simulink model "kre_discrete_observer_wrapper"  (R2026a)
settings: Solver=FixedStepDiscrete  FixedStep=5e-5
settings Model: Creator=hzldx  LastModifiedBy=ASUS
settings HardwareCC: ProdLargestAtomicInteger=Long  ProdLargestAtomicFloat=Double  ProdHWDeviceType=ARM Compatible->ARM Cortex-M  TargetLargestAtomicInteger=Long  TargetLargestAtomicFloat=Double  TargetIntDivRoundTo=Zero  TargetEndianess=LittleEndian  TargetHWDeviceType=ARM Compatible->ARM Cortex-M  ProdEqTarget=off
settings RTWCC: SystemTargetFile=ert.tlc  GenCodeOnly=on  GenerateMakefile=off  Description=Embedded Coder
settings ERTTargetCC: GenerateSampleERTMain=on

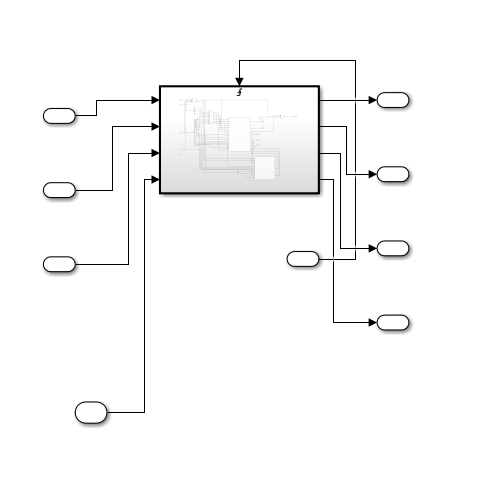
[thumbnail: Simulink's stored preview of the top-level diagram]
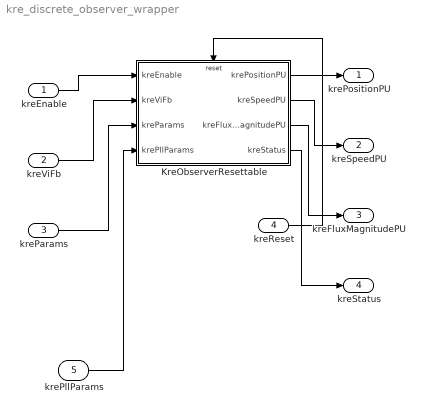
== system kre_discrete_observer_wrapper ==
  kreEnable : Inport  OutDataTypeStr=uint8  PortDimensions=1  SampleTime=5e-5
  kreViFb : Inport  Port=2  OutDataTypeStr=single  PortDimensions=[4 1]  SampleTime=5e-5
  kreParams : Inport  Port=3  OutDataTypeStr=single  PortDimensions=[14 1]  SampleTime=5e-5
  kreReset : Inport  Port=4  OutDataTypeStr=uint8  PortDimensions=1  SampleTime=5e-5
  krePllParams : Inport  Port=5  OutDataTypeStr=single  PortDimensions=[2 1]  SampleTime=5e-5
  KreObserverResettable : Subsystem  TreatAsAtomicUnit=on
  krePositionPU : Outport  OutDataTypeStr=single  PortDimensions=1  SampleTime=5e-5
  kreSpeedPU : Outport  Port=2  OutDataTypeStr=single  PortDimensions=1  SampleTime=5e-5
  kreFluxMagnitudePU : Outport  Port=3  OutDataTypeStr=single  PortDimensions=1  SampleTime=5e-5
  kreStatus : Outport  Port=4  OutDataTypeStr=uint8  PortDimensions=1  SampleTime=5e-5
  wires:
  kreReset/1 -> KreObserverResettable/Reset
  kreEnable/1 -> KreObserverResettable/1(kreEnable)
  kreViFb/1 -> KreObserverResettable/2(kreViFb)
  kreParams/1 -> KreObserverResettable/3(kreParams)
  KreObserverResettable/1(krePositionPU) -> krePositionPU/1
  KreObserverResettable/2(kreSpeedPU) -> kreSpeedPU/1
  KreObserverResettable/3(kreFluxMagnitudePU) -> kreFluxMagnitudePU/1
  KreObserverResettable/4(kreStatus) -> kreStatus/1
  krePllParams/1 -> KreObserverResettable/4(krePllParams)

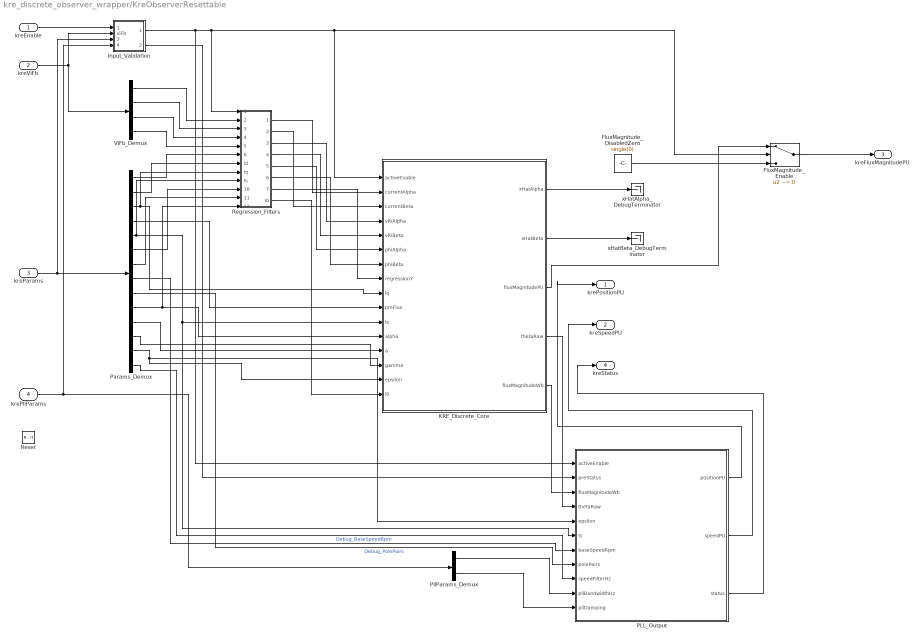
== system kre_discrete_observer_wrapper/KreObserverResettable ==
  kreEnable : Inport  OutDataTypeStr=uint8  PortDimensions=1  SampleTime=5e-5
  kreViFb : Inport  Port=2  OutDataTypeStr=single  PortDimensions=[4 1]  SampleTime=5e-5
  kreParams : Inport  Port=3  OutDataTypeStr=single  PortDimensions=[14 1]  SampleTime=5e-5
  krePllParams : Inport  Port=4  OutDataTypeStr=single  PortDimensions=[2 1]  SampleTime=5e-5
  Reset : ResetPort  DisableCoverage=on
  FluxMagnitude_DisabledZero : Constant  Value=single(0)  OutDataTypeStr=single
  FluxMagnitude_Enable : Switch  Criteria=u2 ~= 0  SaturateOnIntegerOverflow=off  InputSameDT=off
  Input_Validation : Subsystem
  KRE_Discrete_Core : Subsystem
  PLL_Output : Subsystem
  Params_Demux : Demux  Outputs=14
  PllParams_Demux : Demux  Outputs=2
  Regression_Filters : Subsystem
  ViFb_Demux : Demux
  xHatAlpha_DebugTerminator : Terminator
  xHatBeta_DebugTerminator : Terminator
  krePositionPU : Outport  OutDataTypeStr=single  PortDimensions=1  SampleTime=5e-5
  kreSpeedPU : Outport  Port=2  OutDataTypeStr=single  PortDimensions=1  SampleTime=5e-5
  kreFluxMagnitudePU : Outport  Port=3  OutDataTypeStr=single  PortDimensions=1  SampleTime=5e-5
  kreStatus : Outport  Port=4  OutDataTypeStr=uint8  PortDimensions=1  SampleTime=5e-5
  wires:
  Params_Demux/7 -> Regression_Filters/11(baseCurrent)
  Params_Demux/6 -> Regression_Filters/10(baseVoltage)
  Params_Demux/2 -> Regression_Filters/7(ld)
  Params_Demux/1 -> Regression_Filters/6(resistance)
  ViFb_Demux/4 -> Regression_Filters/5(iBetaPU)
  ViFb_Demux/3 -> Regression_Filters/4(iAlphaPU)
  ViFb_Demux/2 -> Regression_Filters/3(vBetaPU)
  ViFb_Demux/1 -> Regression_Filters/2(vAlphaPU)
  kreEnable/1 -> Input_Validation/1(enable)
  kreParams/1 -> Params_Demux/1, Input_Validation/3(params)
  kreViFb/1 -> Input_Validation/2(viFb), ViFb_Demux/1
  KRE_Discrete_Core/2(xHatBeta) -> xHatBeta_DebugTerminator/1
  KRE_Discrete_Core/1(xHatAlpha) -> xHatAlpha_DebugTerminator/1
  Params_Demux/3 -> KRE_Discrete_Core/9(lq), Regression_Filters/8(lq)
  Params_Demux/10 -> KRE_Discrete_Core/12(alpha), Regression_Filters/12(alpha)
  Regression_Filters/1(currentAlpha) -> KRE_Discrete_Core/2(currentAlpha)
  Regression_Filters/2(currentBeta) -> KRE_Discrete_Core/3(currentBeta)
  Regression_Filters/3(vRiAlpha) -> KRE_Discrete_Core/4(vRiAlpha)
  Regression_Filters/4(vRiBeta) -> KRE_Discrete_Core/5(vRiBeta)
  Regression_Filters/5(phiAlpha) -> KRE_Discrete_Core/6(phiAlpha)
  Regression_Filters/6(phiBeta) -> KRE_Discrete_Core/7(phiBeta)
  Regression_Filters/7(regressionY) -> KRE_Discrete_Core/8(regressionY)
  Params_Demux/4 -> KRE_Discrete_Core/10(pmFlux)
  Params_Demux/11 -> KRE_Discrete_Core/13(a)
  Params_Demux/12 -> KRE_Discrete_Core/14(gamma)
  Regression_Filters/8(l0) -> KRE_Discrete_Core/16(l0)
  FluxMagnitude_Enable/1 -> kreFluxMagnitudePU/1
  FluxMagnitude_DisabledZero/1 -> FluxMagnitude_Enable/3
  KRE_Discrete_Core/3(fluxMagnitudePU) -> FluxMagnitude_Enable/1
  PLL_Output/3(status) -> kreStatus/1
  PLL_Output/2(speedPU) -> kreSpeedPU/1
  PLL_Output/1(positionPU) -> krePositionPU/1
  PllParams_Demux/2 -> PLL_Output/11(pllDamping)
  PllParams_Demux/1 -> PLL_Output/10(pllBandwidthHz)
  Params_Demux/14 -> PLL_Output/9(speedFilterHz)
  Params_Demux/9 -> PLL_Output/8(polePairs)  "Debug_PolePairs"
  Params_Demux/8 -> PLL_Output/7(baseSpeedRpm)  "Debug_BaseSpeedRpm"
  KRE_Discrete_Core/4(thetaRaw) -> PLL_Output/4(thetaRaw)
  Input_Validation/2(preStatus) -> PLL_Output/2(preStatus)
  Params_Demux/13 -> KRE_Discrete_Core/15(epsilon), PLL_Output/5(epsilon)
  Params_Demux/5 -> PLL_Output/6(ts), KRE_Discrete_Core/11(ts), Regression_Filters/9(ts)
  Input_Validation/1(activeEnable) -> FluxMagnitude_Enable/2, KRE_Discrete_Core/1(activeEnable), Regression_Filters/1(activeEnable), PLL_Output/1(activeEnable)
  krePllParams/1 -> PllParams_Demux/1, Input_Validation/4(pllParams)
  KRE_Discrete_Core/5(fluxMagnitudeWb) -> PLL_Output/3(fluxMagnitudeWb)

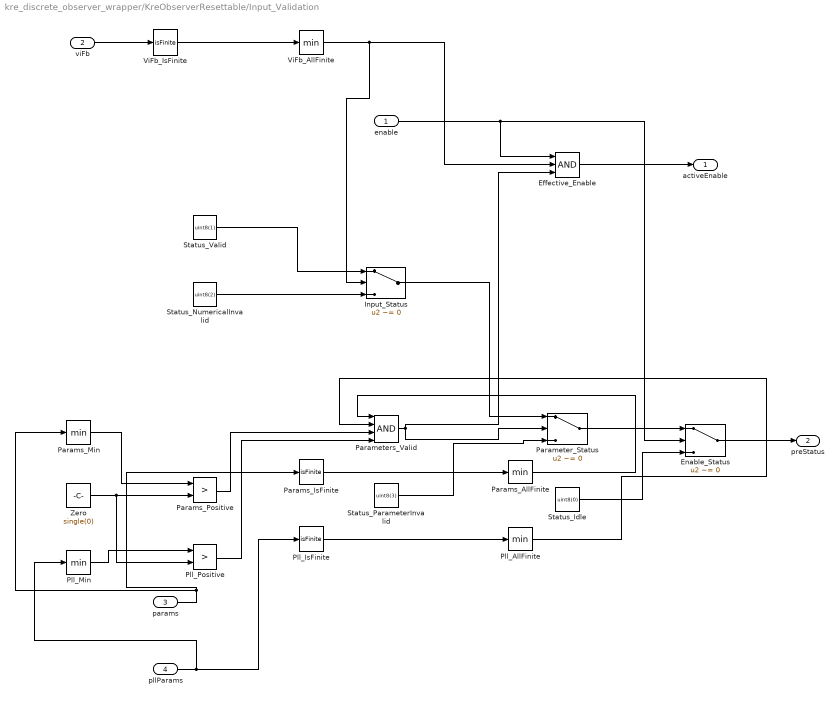
== system kre_discrete_observer_wrapper/KreObserverResettable/Input_Validation ==
  enable : Inport
  viFb : Inport  Port=2
  params : Inport  Port=3
  pllParams : Inport  Port=4
  Effective_Enable : Logic  Inputs=3  IconShape=distinctive  AllPortsSameDT=off  OutDataTypeStr=boolean
  Enable_Status : Switch  Criteria=u2 ~= 0  SaturateOnIntegerOverflow=off  InputSameDT=off
  Input_Status : Switch  Criteria=u2 ~= 0  SaturateOnIntegerOverflow=off  InputSameDT=off
  Parameter_Status : Switch  Criteria=u2 ~= 0  SaturateOnIntegerOverflow=off  InputSameDT=off
  Parameters_Valid : Logic  Inputs=4  IconShape=distinctive  AllPortsSameDT=off  OutDataTypeStr=boolean
  Params_AllFinite : MinMax
  Params_IsFinite : RelationalOperator  Operator=isFinite  OutDataTypeStr=boolean  RndMeth=Simplest  InputSameDT=off
  Params_Min : MinMax
  Params_Positive : RelationalOperator  Operator=>  OutDataTypeStr=boolean  RndMeth=Simplest  InputSameDT=off
  Pll_AllFinite : MinMax
  Pll_IsFinite : RelationalOperator  Operator=isFinite  OutDataTypeStr=boolean  RndMeth=Simplest  InputSameDT=off
  Pll_Min : MinMax
  Pll_Positive : RelationalOperator  Operator=>  OutDataTypeStr=boolean  RndMeth=Simplest  InputSameDT=off
  Status_Idle : Constant  Value=uint8(0)  OutDataTypeStr=uint8
  Status_NumericalInvalid : Constant  Value=uint8(2)  OutDataTypeStr=uint8
  Status_ParameterInvalid : Constant  Value=uint8(3)  OutDataTypeStr=uint8
  Status_Valid : Constant  Value=uint8(1)  OutDataTypeStr=uint8
  ViFb_AllFinite : MinMax
  ViFb_IsFinite : RelationalOperator  Operator=isFinite  OutDataTypeStr=boolean  RndMeth=Simplest  InputSameDT=off
  Zero : Constant  Value=single(0)  OutDataTypeStr=single
  activeEnable : Outport
  preStatus : Outport  Port=2
  wires:
  Enable_Status/1 -> preStatus/1
  Status_Idle/1 -> Enable_Status/3
  Parameter_Status/1 -> Enable_Status/1
  Status_ParameterInvalid/1 -> Parameter_Status/3
  Input_Status/1 -> Parameter_Status/1
  Status_NumericalInvalid/1 -> Input_Status/3
  Status_Valid/1 -> Input_Status/1
  Effective_Enable/1 -> activeEnable/1
  Parameters_Valid/1 -> Effective_Enable/3, Parameter_Status/2
  enable/1 -> Effective_Enable/1, Enable_Status/2
  Pll_Positive/1 -> Parameters_Valid/4
  Params_Positive/1 -> Parameters_Valid/3
  Pll_Min/1 -> Pll_Positive/1
  Zero/1 -> Params_Positive/2, Pll_Positive/2
  Params_Min/1 -> Params_Positive/1
  Pll_IsFinite/1 -> Pll_AllFinite/1
  Params_IsFinite/1 -> Params_AllFinite/1
  ViFb_IsFinite/1 -> ViFb_AllFinite/1
  viFb/1 -> ViFb_IsFinite/1
  params/1 -> Params_IsFinite/1, Params_Min/1
  pllParams/1 -> Pll_IsFinite/1, Pll_Min/1
  Params_AllFinite/1 -> Parameters_Valid/1
  Pll_AllFinite/1 -> Parameters_Valid/2
  ViFb_AllFinite/1 -> Input_Status/2, Effective_Enable/2

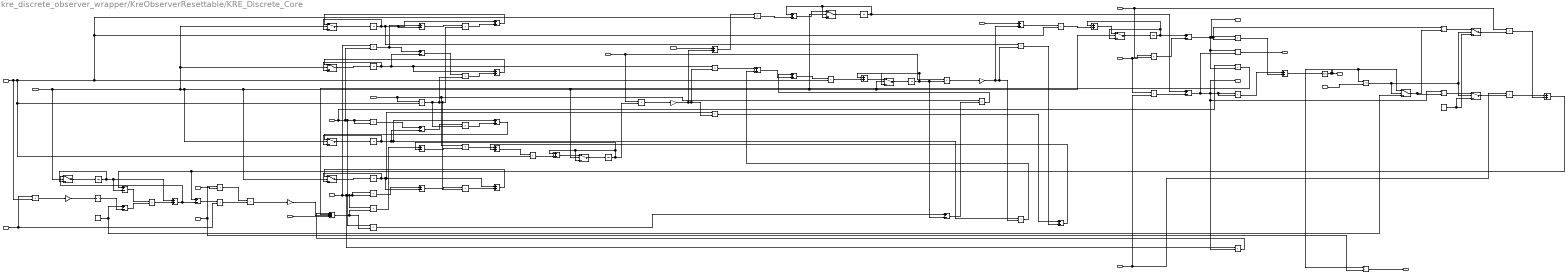
== system kre_discrete_observer_wrapper/KreObserverResettable/KRE_Discrete_Core ==
  activeEnable : Inport
  currentAlpha : Inport  Port=2
  currentBeta : Inport  Port=3
  vRiAlpha : Inport  Port=4
  vRiBeta : Inport  Port=5
  phiAlpha : Inport  Port=6
  phiBeta : Inport  Port=7
  regressionY : Inport  Port=8
  lq : Inport  Port=9
  pmFlux : Inport  Port=10
  ts : Inport  Port=11
  alpha : Inport  Port=12
  a : Inport  Port=13
  gamma : Inport  Port=14
  epsilon : Inport  Port=15
  l0 : Inport  Port=16
  A_Ts : Product
  A_YAlphaError : Product
  A_YBetaError : Product
  ActiveFluxAlpha_Square : Product
  ActiveFluxBeta_Square : Product
  ActiveFlux_Alpha : Sum  Inputs=+-
  ActiveFlux_Beta : Sum  Inputs=+-
  ActiveFlux_Magnitude : Math  Operator=sqrt  SignedPower=on  RndMeth=Zero
  ActiveFlux_NormSquare : Sum
  Alpha_Ts : Product
  CorrectionE_Alpha : Gain  Gain=single(-1)
  CorrectionE_Beta : Gain  Gain=single(-1)
  CurrentDotSigma : Sum
  CurrentDotSigma_Alpha : Product
  CurrentDotSigma_Beta : Product
  Disturbance_Magnitude : Product
  Disturbance_Negative : Gain  Gain=single(-1)
  Exp_NegAlphaTs : Math  SignedPower=on  RndMeth=Zero
  FluxMagnitude_PU : Product  Inputs=*/
  Flux_Above_Epsilon : RelationalOperator  OutDataTypeStr=boolean  RndMeth=Simplest  InputSameDT=off
  Flux_Angle : Trigonometry  Operator=atan2
  GammaY_Alpha : Product
  GammaY_Beta : Product
  H1D : Product
  H1D_Error : Sum  Inputs=+-
  H2D_Correction : Product
  H2D_Error : Sum  Inputs=+-
  H2D_Hold : Switch  Criteria=u2 ~= 0  SaturateOnIntegerOverflow=off  InputSameDT=off
  H2D_Next : Sum
  H2D_State : UnitDelay  InitialCondition=single(0)  SampleTime=-1
  H2_Gain : Sum  Inputs=+-
  LambdaAlpha_Delta : Product
  LambdaAlpha_Derivative : Sum
  LambdaAlpha_Hold : Switch  Criteria=u2 ~= 0  SaturateOnIntegerOverflow=off  InputSameDT=off
  LambdaAlpha_Next : Sum
  LambdaAlpha_State : UnitDelay  InitialCondition=single(0)  SampleTime=-1
  LambdaBeta_Delta : Product
  LambdaBeta_Derivative : Sum
  LambdaBeta_Hold : Switch  Criteria=u2 ~= 0  SaturateOnIntegerOverflow=off  InputSameDT=off
  LambdaBeta_Next : Sum
  LambdaBeta_State : UnitDelay  InitialCondition=single(0)  SampleTime=-1
  Lq_CurrentAlpha : Product
  Lq_CurrentBeta : Product
  Negative_AlphaTs : Gain  Gain=single(-1)
  One : Constant  Value=single(1)  OutDataTypeStr=single
  PhiAlphaBeta : Product
  PhiAlpha_Square : Product
  PhiBeta_Square : Product
  PhiE_Alpha : Product
  PhiE_Beta : Product
  PhiX_Alpha : Product
  PhiX_Beta : Product
  PsiM_L0 : Product
  Q11_Correction : Product
  Q11_EAlpha : Product
  Q11_Hold : Switch  Criteria=u2 ~= 0  SaturateOnIntegerOverflow=off  InputSameDT=off
  Q11_Next : Sum
  Q11_State : UnitDelay  InitialCondition=single(0)  SampleTime=-1
  Q11_TargetMinusState : Sum  Inputs=+-
  Q12_Correction : Product
  Q12_EBeta : Product
  Q12_Hold : Switch  Criteria=u2 ~= 0  SaturateOnIntegerOverflow=off  InputSameDT=off
  Q12_Next : Sum
  Q12_State : UnitDelay  InitialCondition=single(0)  SampleTime=-1
  Q12_TargetMinusState : Sum  Inputs=+-
  Q21_Correction : Product
  Q21_EAlpha : Product
  Q21_Hold : Switch  Criteria=u2 ~= 0  SaturateOnIntegerOverflow=off  InputSameDT=off
  Q21_Next : Sum
  Q21_State : UnitDelay  InitialCondition=single(0)  SampleTime=-1
  Q21_TargetMinusState : Sum  Inputs=+-
  Q22_Correction : Product
  Q22_EBeta : Product
  Q22_Hold : Switch  Criteria=u2 ~= 0  SaturateOnIntegerOverflow=off  InputSameDT=off
  Q22_Next : Sum
  Q22_State : UnitDelay  InitialCondition=single(0)  SampleTime=-1
  Q22_TargetMinusState : Sum  Inputs=+-
  Q_E_Alpha : Sum
  Q_E_Beta : Sum
  Regression_Error : Sum  Inputs=+++-
  Safe_Flux_Magnitude : Switch  Criteria=u2 ~= 0  SaturateOnIntegerOverflow=off  InputSameDT=off
  Sigma_Alpha : Switch  Criteria=u2 ~= 0  SaturateOnIntegerOverflow=off  InputSameDT=off
  Sigma_Alpha_Raw : Product  Inputs=*/
  Sigma_Beta : Switch  Criteria=u2 ~= 0  SaturateOnIntegerOverflow=off  InputSameDT=off
  Sigma_Beta_Raw : Product  Inputs=*/
  YAlpha_Delta : Product
  YAlpha_Derivative : Sum
  YAlpha_Hold : Switch  Criteria=u2 ~= 0  SaturateOnIntegerOverflow=off  InputSameDT=off
  YAlpha_Next : Sum
  YAlpha_State : UnitDelay  InitialCondition=single(0)  SampleTime=-1
  YAlpha_TargetMinusState : Sum  Inputs=+-
  YBeta_Delta : Product
  YBeta_Derivative : Sum
  YBeta_Hold : Switch  Criteria=u2 ~= 0  SaturateOnIntegerOverflow=off  InputSameDT=off
  YBeta_Next : Sum
  YBeta_State : UnitDelay  InitialCondition=single(0)  SampleTime=-1
  YBeta_TargetMinusState : Sum  Inputs=+-
  Zero : Constant  Value=single(0)  OutDataTypeStr=single
  xHatAlpha : Outport
  xHatBeta : Outport  Port=2
  fluxMagnitudePU : Outport  Port=3
  thetaRaw : Outport  Port=4
  fluxMagnitudeWb : Outport  Port=5
  wires:
  Flux_Angle/1 -> thetaRaw/1
  FluxMagnitude_PU/1 -> fluxMagnitudePU/1
  LambdaBeta_Hold/1 -> LambdaBeta_State/1
  LambdaBeta_Next/1 -> LambdaBeta_Hold/1
  LambdaAlpha_Hold/1 -> LambdaAlpha_State/1
  LambdaAlpha_Next/1 -> LambdaAlpha_Hold/1
  LambdaBeta_Delta/1 -> LambdaBeta_Next/2
  LambdaAlpha_Delta/1 -> LambdaAlpha_Next/2
  LambdaBeta_Derivative/1 -> LambdaBeta_Delta/1
  LambdaAlpha_Derivative/1 -> LambdaAlpha_Delta/1
  vRiBeta/1 -> LambdaBeta_Derivative/1
  vRiAlpha/1 -> LambdaAlpha_Derivative/1
  YBeta_Hold/1 -> YBeta_State/1
  YBeta_Next/1 -> YBeta_Hold/1
  YAlpha_Hold/1 -> YAlpha_State/1
  YAlpha_Next/1 -> YAlpha_Hold/1
  YBeta_Delta/1 -> YBeta_Next/2
  YAlpha_Delta/1 -> YAlpha_Next/2
  YBeta_Derivative/1 -> YBeta_Delta/1
  YAlpha_Derivative/1 -> YAlpha_Delta/1
  Q_E_Beta/1 -> YBeta_Derivative/2
  A_YBetaError/1 -> YBeta_Derivative/1
  Q_E_Alpha/1 -> YAlpha_Derivative/2
  A_YAlphaError/1 -> YAlpha_Derivative/1
  YBeta_TargetMinusState/1 -> A_YBetaError/2
  YAlpha_TargetMinusState/1 -> A_YAlphaError/2
  PhiE_Beta/1 -> YBeta_TargetMinusState/1
  PhiE_Alpha/1 -> YAlpha_TargetMinusState/1
  Regression_Error/1 -> PhiE_Alpha/2, PhiE_Beta/2
  Q22_EBeta/1 -> Q_E_Beta/2
  Q21_EAlpha/1 -> Q_E_Beta/1
  Q12_EBeta/1 -> Q_E_Alpha/2
  Q11_EAlpha/1 -> Q_E_Alpha/1
  CorrectionE_Beta/1 -> Q12_EBeta/2, Q22_EBeta/2, LambdaBeta_Derivative/2
  CorrectionE_Alpha/1 -> Q11_EAlpha/2, Q21_EAlpha/2, LambdaAlpha_Derivative/2
  Q22_Hold/1 -> Q22_State/1
  Q22_Next/1 -> Q22_Hold/1
  Q22_Correction/1 -> Q22_Next/2
  Q22_TargetMinusState/1 -> Q22_Correction/1
  Q22_State/1 -> Q22_Next/1, Q22_EBeta/1, Q22_TargetMinusState/2, Q22_Hold/3
  PhiBeta_Square/1 -> Q22_TargetMinusState/1
  Q12_Hold/1 -> Q12_State/1
  Q12_Next/1 -> Q12_Hold/1
  Q12_Correction/1 -> Q12_Next/2
  Q12_TargetMinusState/1 -> Q12_Correction/1
  Q12_State/1 -> Q12_Next/1, Q12_TargetMinusState/2, Q12_EBeta/1, Q12_Hold/3
  Q21_Hold/1 -> Q21_State/1
  Q21_Next/1 -> Q21_Hold/1
  Q21_Correction/1 -> Q21_Next/2
  Q21_TargetMinusState/1 -> Q21_Correction/1
  Q21_State/1 -> Q21_Next/1, Q21_EAlpha/1, Q21_TargetMinusState/2, Q21_Hold/3
  PhiAlphaBeta/1 -> Q21_TargetMinusState/1, Q12_TargetMinusState/1
  Q11_Hold/1 -> Q11_State/1
  Q11_Next/1 -> Q11_Hold/1
  Q11_Correction/1 -> Q11_Next/2
  A_Ts/1 -> Q11_Correction/2, Q12_Correction/2, Q21_Correction/2, Q22_Correction/2
  Q11_TargetMinusState/1 -> Q11_Correction/1
  Q11_State/1 -> Q11_Next/1, Q11_EAlpha/1, Q11_TargetMinusState/2, Q11_Hold/3
  PhiAlpha_Square/1 -> Q11_TargetMinusState/1
  a/1 -> A_YAlphaError/1, A_YBetaError/1, A_Ts/1
  GammaY_Beta/1 -> CorrectionE_Beta/1
  GammaY_Alpha/1 -> CorrectionE_Alpha/1
  YBeta_State/1 -> YBeta_TargetMinusState/2, GammaY_Beta/2, YBeta_Next/1, YBeta_Hold/3
  YAlpha_State/1 -> YAlpha_Next/1, YAlpha_Hold/3, YAlpha_TargetMinusState/2, GammaY_Alpha/2
  gamma/1 -> GammaY_Alpha/1, GammaY_Beta/1
  regressionY/1 -> Regression_Error/4
  Disturbance_Negative/1 -> Regression_Error/3
  PhiX_Beta/1 -> Regression_Error/2
  PhiX_Alpha/1 -> Regression_Error/1
  phiBeta/1 -> PhiBeta_Square/2, PhiBeta_Square/1, PhiE_Beta/1, PhiAlphaBeta/2, PhiX_Beta/1
  phiAlpha/1 -> PhiAlpha_Square/1, PhiAlpha_Square/2, PhiE_Alpha/1, PhiX_Alpha/1, PhiAlphaBeta/1
  Disturbance_Magnitude/1 -> Disturbance_Negative/1
  H1D/1 -> Disturbance_Magnitude/2
  PsiM_L0/1 -> Disturbance_Magnitude/1
  l0/1 -> PsiM_L0/2
  pmFlux/1 -> PsiM_L0/1, FluxMagnitude_PU/2
  H1D_Error/1 -> H1D/1
  H2D_Hold/1 -> H2D_State/1
  activeEnable/1 -> YBeta_Hold/2, LambdaBeta_Hold/2, LambdaAlpha_Hold/2, YAlpha_Hold/2, Q11_Hold/2, Q22_Hold/2, Q21_Hold/2, Q12_Hold/2, H2D_Hold/2
  H2D_Next/1 -> H2D_Hold/1, H1D_Error/2
  H2D_Correction/1 -> H2D_Next/2
  H2_Gain/1 -> H2D_Correction/2
  H2D_Error/1 -> H2D_Correction/1
  H2D_State/1 -> H2D_Error/2, H2D_Next/1, H2D_Hold/3
  CurrentDotSigma/1 -> H2D_Error/1, H1D_Error/1
  CurrentDotSigma_Beta/1 -> CurrentDotSigma/2
  CurrentDotSigma_Alpha/1 -> CurrentDotSigma/1
  Sigma_Beta/1 -> CurrentDotSigma_Beta/2
  Sigma_Alpha/1 -> CurrentDotSigma_Alpha/2
  Sigma_Beta_Raw/1 -> Sigma_Beta/1
  Zero/1 -> Sigma_Alpha/3, Sigma_Beta/3
  Sigma_Alpha_Raw/1 -> Sigma_Alpha/1
  Safe_Flux_Magnitude/1 -> Sigma_Alpha_Raw/2, Sigma_Beta_Raw/2
  Flux_Above_Epsilon/1 -> Sigma_Alpha/2, Sigma_Beta/2, Safe_Flux_Magnitude/2
  epsilon/1 -> Flux_Above_Epsilon/2
  ActiveFlux_NormSquare/1 -> ActiveFlux_Magnitude/1
  ActiveFluxBeta_Square/1 -> ActiveFlux_NormSquare/2
  ActiveFluxAlpha_Square/1 -> ActiveFlux_NormSquare/1
  ActiveFlux_Beta/1 -> Flux_Angle/1, PhiX_Beta/2, Sigma_Beta_Raw/1, ActiveFluxBeta_Square/2, ActiveFluxBeta_Square/1, xHatBeta/1
  ActiveFlux_Alpha/1 -> PhiX_Alpha/2, Sigma_Alpha_Raw/1, ActiveFluxAlpha_Square/2, ActiveFluxAlpha_Square/1, xHatAlpha/1, Flux_Angle/2
  Lq_CurrentBeta/1 -> ActiveFlux_Beta/2
  LambdaBeta_State/1 -> LambdaBeta_Next/1, LambdaBeta_Hold/3, ActiveFlux_Beta/1
  Lq_CurrentAlpha/1 -> ActiveFlux_Alpha/2
  LambdaAlpha_State/1 -> LambdaAlpha_Next/1, LambdaAlpha_Hold/3, ActiveFlux_Alpha/1
  currentBeta/1 -> Lq_CurrentBeta/2, CurrentDotSigma_Beta/1
  currentAlpha/1 -> Lq_CurrentAlpha/2, CurrentDotSigma_Alpha/1
  lq/1 -> Lq_CurrentAlpha/1, Lq_CurrentBeta/1
  Exp_NegAlphaTs/1 -> H2_Gain/2
  One/1 -> H2_Gain/1, Safe_Flux_Magnitude/3
  Negative_AlphaTs/1 -> Exp_NegAlphaTs/1
  Alpha_Ts/1 -> Negative_AlphaTs/1
  ts/1 -> A_Ts/2, YAlpha_Delta/2, LambdaAlpha_Delta/2, LambdaBeta_Delta/2, YBeta_Delta/2, Alpha_Ts/2
  alpha/1 -> Alpha_Ts/1, H1D/2
  ActiveFlux_Magnitude/1 -> Safe_Flux_Magnitude/1, Flux_Above_Epsilon/1, fluxMagnitudeWb/1, FluxMagnitude_PU/1

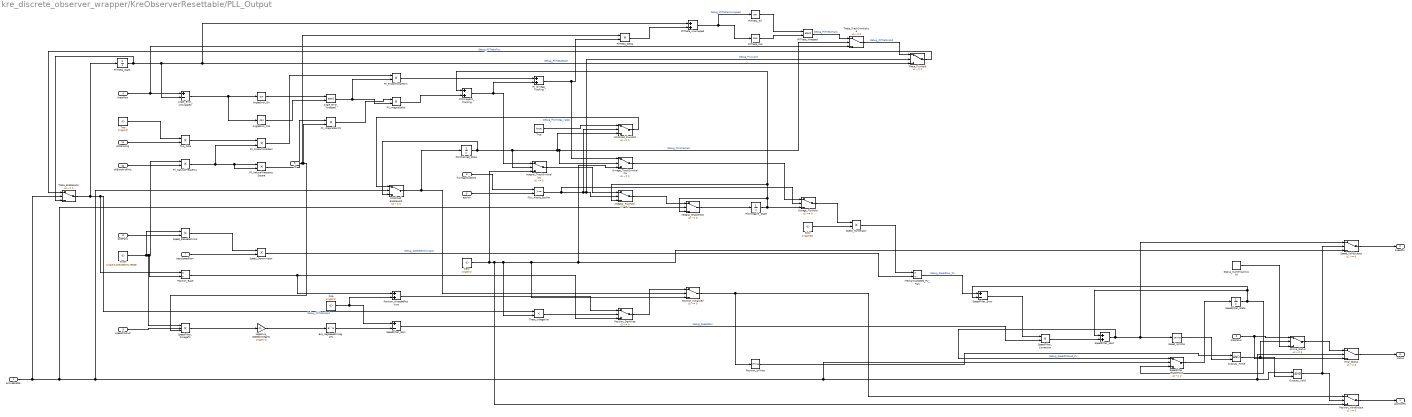
== system kre_discrete_observer_wrapper/KreObserverResettable/PLL_Output ==
  activeEnable : Inport
  preStatus : Inport  Port=2
  fluxMagnitudeWb : Inport  Port=3
  thetaRaw : Inport  Port=4
  epsilon : Inport  Port=5
  ts : Inport  Port=6
  baseSpeedRpm : Inport  Port=7
  polePairs : Inport  Port=8
  speedFilterHz : Inport  Port=9
  pllBandwidthHz : Inport  Port=10
  pllDamping : Inport  Port=11
  Active_Status : Switch  Criteria=u2 ~= 0  SaturateOnIntegerOverflow=off  InputSameDT=off
  AngleError_Cos : Trigonometry  Operator=cos
  AngleError_Sin : Trigonometry
  Angle_Error_Unwrapped : Sum  Inputs=+-
  Angle_Error_Wrapped : Trigonometry  Operator=atan2
  Exp_NegSpeedOmegaTs : Math  SignedPower=on  RndMeth=Zero
  Final_Status : Switch  Criteria=u2 ~= 0  SaturateOnIntegerOverflow=off  InputSameDT=off
  Flux_Above_Epsilon : RelationalOperator  OutDataTypeStr=boolean  RndMeth=Simplest  InputSameDT=off
  Initialized_EnableHold : Switch  Criteria=u2 ~= 0  SaturateOnIntegerOverflow=off  InputSameDT=off
  Initialized_FluxHold : Switch  Criteria=u2 ~= 0  SaturateOnIntegerOverflow=off  InputSameDT=off
  Integral_EnableHold : Switch  Criteria=u2 ~= 0  SaturateOnIntegerOverflow=off  InputSameDT=off
  Integral_FluxHold : Switch  Criteria=u2 ~= 0  SaturateOnIntegerOverflow=off  InputSameDT=off
  Integral_TrackOrInitialize : Switch  Criteria=u2 ~= 0  SaturateOnIntegerOverflow=off  InputSameDT=off
  MechanicalSpeed_PU_Raw : Product  Inputs=*/
  Negative_SpeedOmegaTs : Gain  Gain=single(-1)
  Omega_FluxHold : Switch  Criteria=u2 ~= 0  SaturateOnIntegerOverflow=off  InputSameDT=off
  Omega_TrackOrInitialize : Switch  Criteria=u2 ~= 0  SaturateOnIntegerOverflow=off  InputSameDT=off
  One : Constant  Value=single(1)  OutDataTypeStr=single
  Outputs_Finite : Logic  IconShape=distinctive  AllPortsSameDT=off  OutDataTypeStr=boolean
  Outputs_Valid : Logic  IconShape=distinctive  AllPortsSameDT=off  OutDataTypeStr=boolean
  PllInitialized_State : UnitDelay  InitialCondition=false  SampleTime=-1
  PllOmegaInt_State : UnitDelay  InitialCondition=single(0)  SampleTime=-1
  PllOmegaInt_Tracking : Sum
  PllTheta_Cos : Trigonometry  Operator=cos
  PllTheta_Delta : Product
  PllTheta_Sin : Trigonometry
  PllTheta_State : UnitDelay  InitialCondition=single(0)  SampleTime=-1
  PllTheta_Unwrapped : Sum
  PllTheta_Wrapped : Trigonometry  Operator=atan2
  Pll_IntegralDelta : Product
  Pll_IntegralGainTs : Product
  Pll_NaturalFrequency : Product
  Pll_NaturalFrequencySquare : Product
  Pll_Omega_Tracking : Sum
  Pll_ProportionalGain : Product
  Pll_ProportionalTerm : Product
  Position_Base : Product  Inputs=*/
  Position_Initialized : Switch  Criteria=u2 ~= 0  SaturateOnIntegerOverflow=off  InputSameDT=off
  Position_IsFinite : RelationalOperator  Operator=isFinite  OutDataTypeStr=boolean  RndMeth=Simplest  InputSameDT=off
  Position_SignWrap : Switch  Criteria=u2 ~= 0  SaturateOnIntegerOverflow=off  InputSameDT=off
  Position_ValidOutput : Switch  Criteria=u2 ~= 0  SaturateOnIntegerOverflow=off  InputSameDT=off
  Position_WrappedPositive : Sum
  Sixty : Constant  Value=single(60)  OutDataTypeStr=single
  SpeedFilter_Correction : Product
  SpeedFilter_EnableHold : Switch  Criteria=u2 ~= 0  SaturateOnIntegerOverflow=off  InputSameDT=off
  SpeedFilter_Error : Sum  Inputs=+-
  SpeedFilter_Gain : Sum  Inputs=+-
  SpeedFilter_Next : Sum
  SpeedFilter_OmegaTs : Product  Inputs=***
  SpeedFilter_State : UnitDelay  InitialCondition=single(0)  SampleTime=-1
  Speed_BaseElectrical : Product
  Speed_Denominator : Product
  Speed_IsFinite : RelationalOperator  Operator=isFinite  OutDataTypeStr=boolean  RndMeth=Simplest  InputSameDT=off
  Speed_Numerator : Product
  Speed_ValidOutput : Switch  Criteria=u2 ~= 0  SaturateOnIntegerOverflow=off  InputSameDT=off
  Status_NumericalInvalid : Constant  Value=uint8(2)  OutDataTypeStr=uint8
  Theta_EnableHold : Switch  Criteria=u2 ~= 0  SaturateOnIntegerOverflow=off  InputSameDT=off
  Theta_FluxHold : Switch  Criteria=u2 ~= 0  SaturateOnIntegerOverflow=off  InputSameDT=off
  Theta_IsNegative : RelationalOperator  Operator=<  OutDataTypeStr=boolean  RndMeth=Simplest  InputSameDT=off
  Theta_TrackOrInitialize : Switch  Criteria=u2 ~= 0  SaturateOnIntegerOverflow=off  InputSameDT=off
  True : Constant  Value=true  OutDataTypeStr=boolean
  Two : Constant  Value=single(2)  OutDataTypeStr=single
  TwoPi : Constant  Value=single(6.283185307179586)  OutDataTypeStr=single
  Two_Zeta : Product
  Zero : Constant  Value=single(0)  OutDataTypeStr=single
  positionPU : Outport
  speedPU : Outport  Port=2
  status : Outport  Port=3
  wires:
  Final_Status/1 -> status/1
  Speed_ValidOutput/1 -> speedPU/1
  Position_ValidOutput/1 -> positionPU/1
  Active_Status/1 -> Final_Status/1
  Status_NumericalInvalid/1 -> Active_Status/3
  preStatus/1 -> Active_Status/1, Final_Status/3
  Outputs_Valid/1 -> Position_ValidOutput/2, Speed_ValidOutput/2
  Outputs_Finite/1 -> Outputs_Valid/2, Active_Status/2
  Speed_IsFinite/1 -> Outputs_Finite/2
  Position_IsFinite/1 -> Outputs_Finite/1
  Position_Initialized/1 -> Position_IsFinite/1, Position_ValidOutput/1
  Position_SignWrap/1 -> Position_Initialized/1
  Theta_IsNegative/1 -> Position_SignWrap/2
  Position_WrappedPositive/1 -> Position_SignWrap/1
  Position_Base/1 -> Position_WrappedPositive/1, Position_SignWrap/3
  SpeedFilter_EnableHold/1 -> SpeedFilter_State/1
  SpeedFilter_Next/1 -> Speed_IsFinite/1, Speed_ValidOutput/1, SpeedFilter_EnableHold/1  "Debug_SpeedFiltered_PU"
  SpeedFilter_Correction/1 -> SpeedFilter_Next/2
  SpeedFilter_Gain/1 -> SpeedFilter_Correction/2  "Debug_SpeedGain"
  SpeedFilter_Error/1 -> SpeedFilter_Correction/1
  SpeedFilter_State/1 -> SpeedFilter_Error/2, SpeedFilter_Next/1, SpeedFilter_EnableHold/3
  MechanicalSpeed_PU_Raw/1 -> SpeedFilter_Error/1  "Debug_SpeedRaw_PU"
  Exp_NegSpeedOmegaTs/1 -> SpeedFilter_Gain/2
  One/1 -> SpeedFilter_Gain/1, Position_WrappedPositive/2
  Negative_SpeedOmegaTs/1 -> Exp_NegSpeedOmegaTs/1
  SpeedFilter_OmegaTs/1 -> Negative_SpeedOmegaTs/1
  speedFilterHz/1 -> SpeedFilter_OmegaTs/2
  Speed_Denominator/1 -> MechanicalSpeed_PU_Raw/2  "Debug_SpeedDenominator"
  Speed_Numerator/1 -> MechanicalSpeed_PU_Raw/1
  baseSpeedRpm/1 -> Speed_Denominator/2
  Speed_BaseElectrical/1 -> Speed_Denominator/1
  polePairs/1 -> Speed_BaseElectrical/2
  Sixty/1 -> Speed_Numerator/2
  Omega_FluxHold/1 -> Speed_Numerator/1
  Initialized_EnableHold/1 -> PllInitialized_State/1, Position_Initialized/2
  Initialized_FluxHold/1 -> Initialized_EnableHold/1
  Integral_EnableHold/1 -> PllOmegaInt_State/1
  Integral_FluxHold/1 -> Integral_EnableHold/1
  Theta_EnableHold/1 -> Position_Base/1, Theta_IsNegative/1, PllTheta_State/1  "Debug_PllThetaNext"
  activeEnable/1 -> Outputs_Valid/1, Final_Status/2, SpeedFilter_EnableHold/2, Initialized_EnableHold/2, Integral_EnableHold/2, Theta_EnableHold/2
  Theta_FluxHold/1 -> Theta_EnableHold/1  "Debug_PllThetaFlux"
  True/1 -> Initialized_FluxHold/1
  Omega_TrackOrInitialize/1 -> Omega_FluxHold/1
  Integral_TrackOrInitialize/1 -> Integral_FluxHold/1
  Flux_Above_Epsilon/1 -> Theta_FluxHold/2, Integral_FluxHold/2, Initialized_FluxHold/2, Omega_FluxHold/2  "Debug_FluxValid"
  Theta_TrackOrInitialize/1 -> Theta_FluxHold/1  "Debug_PllThetaValid"
  Zero/1 -> Omega_TrackOrInitialize/3, Speed_ValidOutput/3, Position_Initialized/3, Theta_IsNegative/2, Position_ValidOutput/3, Integral_TrackOrInitialize/3
  PllInitialized_State/1 -> Theta_TrackOrInitialize/2, Omega_TrackOrInitialize/2, Initialized_FluxHold/3, Integral_TrackOrInitialize/2, Initialized_EnableHold/3  "Debug_PllInitialized"
  PllTheta_Wrapped/1 -> Theta_TrackOrInitialize/1  "Debug_PllThetaTrack"
  PllTheta_Cos/1 -> PllTheta_Wrapped/2
  PllTheta_Sin/1 -> PllTheta_Wrapped/1
  PllTheta_Unwrapped/1 -> PllTheta_Sin/1, PllTheta_Cos/1  "Debug_PllThetaUnwrapped"
  PllTheta_Delta/1 -> PllTheta_Unwrapped/2
  Pll_Omega_Tracking/1 -> PllTheta_Delta/2, Omega_TrackOrInitialize/1  "Debug_PllOmega_radps"
  PllOmegaInt_Tracking/1 -> Pll_Omega_Tracking/2, Integral_TrackOrInitialize/1
  Pll_ProportionalTerm/1 -> Pll_Omega_Tracking/1
  Pll_ProportionalGain/1 -> Pll_ProportionalTerm/1
  Two_Zeta/1 -> Pll_ProportionalGain/1
  pllDamping/1 -> Two_Zeta/2
  Two/1 -> Two_Zeta/1
  Pll_IntegralDelta/1 -> PllOmegaInt_Tracking/2
  PllOmegaInt_State/1 -> PllOmegaInt_Tracking/1, Integral_FluxHold/3, Integral_EnableHold/3, Omega_FluxHold/3
  Angle_Error_Wrapped/1 -> Pll_IntegralDelta/2, Pll_ProportionalTerm/2
  Pll_IntegralGainTs/1 -> Pll_IntegralDelta/1
  Pll_NaturalFrequencySquare/1 -> Pll_IntegralGainTs/1
  Pll_NaturalFrequency/1 -> Pll_NaturalFrequencySquare/1, Pll_NaturalFrequencySquare/2, Pll_ProportionalGain/2
  pllBandwidthHz/1 -> Pll_NaturalFrequency/2
  TwoPi/1 -> Pll_NaturalFrequency/1, Position_Base/2, SpeedFilter_OmegaTs/1, Speed_BaseElectrical/1
  AngleError_Cos/1 -> Angle_Error_Wrapped/2
  AngleError_Sin/1 -> Angle_Error_Wrapped/1
  Angle_Error_Unwrapped/1 -> AngleError_Sin/1, AngleError_Cos/1
  PllTheta_State/1 -> PllTheta_Unwrapped/1, Theta_FluxHold/3, Angle_Error_Unwrapped/2, Theta_EnableHold/3  "Debug_PllThetaState"
  thetaRaw/1 -> Theta_TrackOrInitialize/3, Angle_Error_Unwrapped/1
  epsilon/1 -> Flux_Above_Epsilon/2
  fluxMagnitudeWb/1 -> Flux_Above_Epsilon/1
  ts/1 -> SpeedFilter_OmegaTs/3, Pll_IntegralGainTs/2, PllTheta_Delta/1

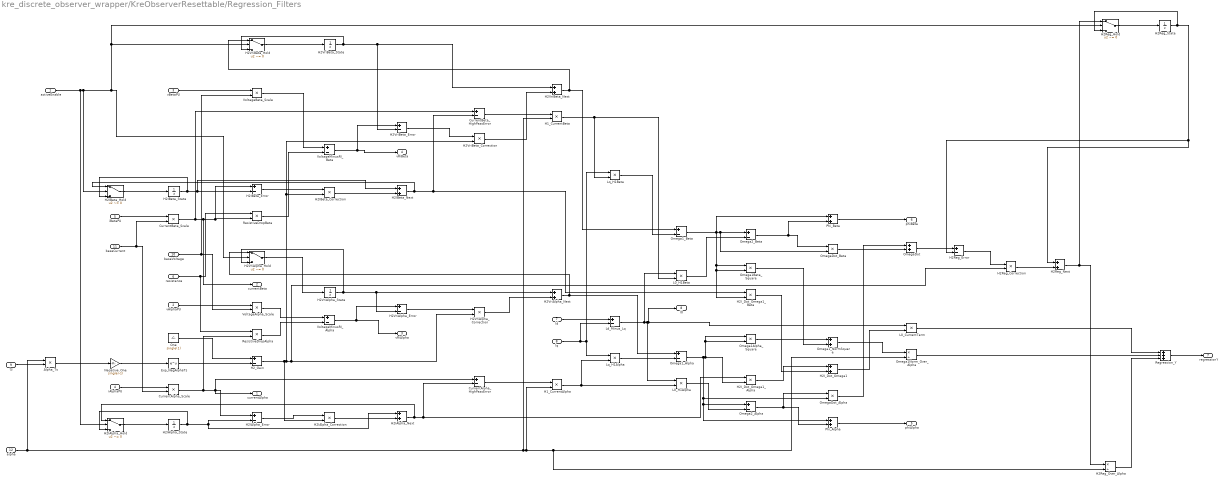
== system kre_discrete_observer_wrapper/KreObserverResettable/Regression_Filters ==
  activeEnable : Inport
  vAlphaPU : Inport  Port=2
  vBetaPU : Inport  Port=3
  iAlphaPU : Inport  Port=4
  iBetaPU : Inport  Port=5
  resistance : Inport  Port=6
  ld : Inport  Port=7
  lq : Inport  Port=8
  ts : Inport  Port=9
  baseVoltage : Inport  Port=10
  baseCurrent : Inport  Port=11
  alpha : Inport  Port=12
  Alpha_Ts : Product
  CurrentAlpha_HighPassError : Sum  Inputs=+-
  CurrentAlpha_Scale : Product
  CurrentBeta_HighPassError : Sum  Inputs=+-
  CurrentBeta_Scale : Product
  Exp_NegAlphaTs : Math  SignedPower=on  RndMeth=Zero
  H1_CurrentAlpha : Product
  H1_CurrentBeta : Product
  H2IAlpha_Correction : Product
  H2IAlpha_Error : Sum  Inputs=+-
  H2IAlpha_Hold : Switch  Criteria=u2 ~= 0  SaturateOnIntegerOverflow=off  InputSameDT=off
  H2IAlpha_Next : Sum
  H2IAlpha_State : UnitDelay  InitialCondition=single(0)  SampleTime=-1
  H2IBeta_Correction : Product
  H2IBeta_Error : Sum  Inputs=+-
  H2IBeta_Hold : Switch  Criteria=u2 ~= 0  SaturateOnIntegerOverflow=off  InputSameDT=off
  H2IBeta_Next : Sum
  H2IBeta_State : UnitDelay  InitialCondition=single(0)  SampleTime=-1
  H2I_Dot_Omega1 : Sum
  H2I_Dot_Omega1_Alpha : Product
  H2I_Dot_Omega1_Beta : Product
  H2Reg_Correction : Product
  H2Reg_Error : Sum  Inputs=+-
  H2Reg_Hold : Switch  Criteria=u2 ~= 0  SaturateOnIntegerOverflow=off  InputSameDT=off
  H2Reg_Next : Sum
  H2Reg_Over_Alpha : Product  Inputs=*/
  H2Reg_State : UnitDelay  InitialCondition=single(0)  SampleTime=-1
  H2VriAlpha_Correction : Product
  H2VriAlpha_Error : Sum  Inputs=+-
  H2VriAlpha_Hold : Switch  Criteria=u2 ~= 0  SaturateOnIntegerOverflow=off  InputSameDT=off
  H2VriAlpha_Next : Sum
  H2VriAlpha_State : UnitDelay  InitialCondition=single(0)  SampleTime=-1
  H2VriBeta_Correction : Product
  H2VriBeta_Error : Sum  Inputs=+-
  H2VriBeta_Hold : Switch  Criteria=u2 ~= 0  SaturateOnIntegerOverflow=off  InputSameDT=off
  H2VriBeta_Next : Sum
  H2VriBeta_State : UnitDelay  InitialCondition=single(0)  SampleTime=-1
  H2_Gain : Sum  Inputs=+-
  L0_CurrentTerm : Product
  L0_H1Alpha : Product
  L0_H1Beta : Product
  Ld_Minus_Lq : Sum  Inputs=+-
  Lq_H1Alpha : Product
  Lq_H1Beta : Product
  Negative_One : Gain  Gain=single(-1)
  Omega1Alpha_Square : Product
  Omega1Beta_Square : Product
  Omega1Norm_Over_Alpha : Product  Inputs=*/
  Omega1_Alpha : Sum  Inputs=+-
  Omega1_Beta : Sum  Inputs=+-
  Omega1_NormSquare : Sum
  Omega2_Alpha : Sum  Inputs=+-
  Omega2_Beta : Sum  Inputs=+-
  OmegaDot : Sum
  OmegaDot_Alpha : Product
  OmegaDot_Beta : Product
  One : Constant  Value=single(1)  OutDataTypeStr=single
  Phi_Alpha : Sum
  Phi_Beta : Sum
  Regression_Y : Sum  Inputs=+++
  ResistiveDropAlpha : Product
  ResistiveDropBeta : Product
  VoltageAlpha_Scale : Product
  VoltageBeta_Scale : Product
  VoltageMinusRI_Alpha : Sum  Inputs=+-
  VoltageMinusRI_Beta : Sum  Inputs=+-
  currentAlpha : Outport
  currentBeta : Outport  Port=2
  vRiAlpha : Outport  Port=3
  vRiBeta : Outport  Port=4
  phiAlpha : Outport  Port=5
  phiBeta : Outport  Port=6
  regressionY : Outport  Port=7
  l0 : Outport  Port=8
  wires:
  Regression_Y/1 -> regressionY/1
  Phi_Beta/1 -> phiBeta/1
  Phi_Alpha/1 -> phiAlpha/1
  H2Reg_Over_Alpha/1 -> Regression_Y/3
  Omega1Norm_Over_Alpha/1 -> Regression_Y/2
  L0_CurrentTerm/1 -> Regression_Y/1
  Omega1_NormSquare/1 -> Omega1Norm_Over_Alpha/1
  Omega1Beta_Square/1 -> Omega1_NormSquare/2
  Omega1Alpha_Square/1 -> Omega1_NormSquare/1
  H2I_Dot_Omega1/1 -> L0_CurrentTerm/2
  H2I_Dot_Omega1_Beta/1 -> H2I_Dot_Omega1/2
  H2I_Dot_Omega1_Alpha/1 -> H2I_Dot_Omega1/1
  H2Reg_Hold/1 -> H2Reg_State/1
  H2Reg_Next/1 -> H2Reg_Hold/1, H2Reg_Over_Alpha/1
  H2Reg_Correction/1 -> H2Reg_Next/2
  H2Reg_Error/1 -> H2Reg_Correction/1
  H2Reg_State/1 -> H2Reg_Error/2, H2Reg_Next/1, H2Reg_Hold/3
  OmegaDot/1 -> H2Reg_Error/1
  OmegaDot_Beta/1 -> OmegaDot/2
  OmegaDot_Alpha/1 -> OmegaDot/1
  Omega2_Beta/1 -> Phi_Beta/2, OmegaDot_Beta/1
  Omega2_Alpha/1 -> Phi_Alpha/2, OmegaDot_Alpha/1
  L0_H1Beta/1 -> Omega2_Beta/2
  Omega1_Beta/1 -> H2I_Dot_Omega1_Beta/2, Omega1Beta_Square/2, Omega1Beta_Square/1, Omega2_Beta/1, OmegaDot_Beta/2, Phi_Beta/1
  L0_H1Alpha/1 -> Omega2_Alpha/2
  Omega1_Alpha/1 -> Phi_Alpha/1, Omega2_Alpha/1, OmegaDot_Alpha/2, Omega1Alpha_Square/1, Omega1Alpha_Square/2, H2I_Dot_Omega1_Alpha/2
  Ld_Minus_Lq/1 -> L0_CurrentTerm/1, l0/1, L0_H1Alpha/1, L0_H1Beta/1
  Lq_H1Beta/1 -> Omega1_Beta/2
  Lq_H1Alpha/1 -> Omega1_Alpha/2
  H1_CurrentBeta/1 -> Lq_H1Beta/2, L0_H1Beta/2
  H1_CurrentAlpha/1 -> Lq_H1Alpha/2, L0_H1Alpha/2
  CurrentBeta_HighPassError/1 -> H1_CurrentBeta/1
  CurrentAlpha_HighPassError/1 -> H1_CurrentAlpha/1
  H2IBeta_Hold/1 -> H2IBeta_State/1
  H2IBeta_Next/1 -> CurrentBeta_HighPassError/2, H2I_Dot_Omega1_Beta/1, H2IBeta_Hold/1
  H2IBeta_Correction/1 -> H2IBeta_Next/2
  H2IBeta_Error/1 -> H2IBeta_Correction/1
  H2IBeta_State/1 -> H2IBeta_Error/2, H2IBeta_Next/1, H2IBeta_Hold/3
  H2IAlpha_Hold/1 -> H2IAlpha_State/1
  H2IAlpha_Next/1 -> CurrentAlpha_HighPassError/2, H2I_Dot_Omega1_Alpha/1, H2IAlpha_Hold/1
  H2IAlpha_Correction/1 -> H2IAlpha_Next/2
  H2IAlpha_Error/1 -> H2IAlpha_Correction/1
  H2IAlpha_State/1 -> H2IAlpha_Next/1, H2IAlpha_Error/2, H2IAlpha_Hold/3
  H2VriBeta_Hold/1 -> H2VriBeta_State/1
  H2VriBeta_Next/1 -> H2VriBeta_Hold/1, Omega1_Beta/1
  H2VriBeta_Correction/1 -> H2VriBeta_Next/2
  H2VriBeta_Error/1 -> H2VriBeta_Correction/1
  H2VriBeta_State/1 -> H2VriBeta_Error/2, H2VriBeta_Next/1, H2VriBeta_Hold/3
  VoltageMinusRI_Beta/1 -> H2VriBeta_Error/1, vRiBeta/1
  H2VriAlpha_Hold/1 -> H2VriAlpha_State/1
  activeEnable/1 -> H2VriBeta_Hold/2, H2Reg_Hold/2, H2VriAlpha_Hold/2, H2IBeta_Hold/2, H2IAlpha_Hold/2
  H2VriAlpha_Next/1 -> Omega1_Alpha/1, H2VriAlpha_Hold/1
  H2VriAlpha_Correction/1 -> H2VriAlpha_Next/2
  H2_Gain/1 -> H2VriAlpha_Correction/2, H2Reg_Correction/2, H2VriBeta_Correction/2, H2IBeta_Correction/2, H2IAlpha_Correction/2
  H2VriAlpha_Error/1 -> H2VriAlpha_Correction/1
  H2VriAlpha_State/1 -> H2VriAlpha_Error/2, H2VriAlpha_Next/1, H2VriAlpha_Hold/3
  VoltageMinusRI_Alpha/1 -> H2VriAlpha_Error/1, vRiAlpha/1
  Exp_NegAlphaTs/1 -> H2_Gain/2
  One/1 -> H2_Gain/1
  Negative_One/1 -> Exp_NegAlphaTs/1
  Alpha_Ts/1 -> Negative_One/1
  ts/1 -> Alpha_Ts/2
  alpha/1 -> Omega1Norm_Over_Alpha/2, H2Reg_Over_Alpha/2, H1_CurrentAlpha/2, H1_CurrentBeta/2, Alpha_Ts/1
  lq/1 -> Lq_H1Alpha/1, Lq_H1Beta/1, Ld_Minus_Lq/2
  ld/1 -> Ld_Minus_Lq/1
  ResistiveDropBeta/1 -> VoltageMinusRI_Beta/2
  VoltageBeta_Scale/1 -> VoltageMinusRI_Beta/1
  ResistiveDropAlpha/1 -> VoltageMinusRI_Alpha/2
  VoltageAlpha_Scale/1 -> VoltageMinusRI_Alpha/1
  CurrentBeta_Scale/1 -> ResistiveDropBeta/2, H2IBeta_Error/1, currentBeta/1, CurrentBeta_HighPassError/1
  CurrentAlpha_Scale/1 -> H2IAlpha_Error/1, CurrentAlpha_HighPassError/1, currentAlpha/1, ResistiveDropAlpha/2
  resistance/1 -> ResistiveDropAlpha/1, ResistiveDropBeta/1
  vBetaPU/1 -> VoltageBeta_Scale/1
  baseVoltage/1 -> VoltageAlpha_Scale/2, VoltageBeta_Scale/2
  vAlphaPU/1 -> VoltageAlpha_Scale/1
  iBetaPU/1 -> CurrentBeta_Scale/1
  baseCurrent/1 -> CurrentAlpha_Scale/2, CurrentBeta_Scale/2
  iAlphaPU/1 -> CurrentAlpha_Scale/1
